simulink model "pacemaker_simulation"  (R2023b)
settings: Solver=FixedStepAuto  StartTime=0.0  StopTime=inf  FixedStep=1e-3  RelTol=1e-3  EnableMultiTasking=on
undefined symbols (not defined in the file): D0, D1, D10, D11, D12, D13, D2, D3, D4, D5, D6, D7, D8, D9, PTA0, PTA1, PTA2, PTB23, PTB9, PTC16, PTC17, PTC2, PTC3, PTC4, PTD0, PTD1, PTD2, PTD3
libraries: frdmk64flib x14
settings Model: ExtModeTrigDuration=5  Creator=stivb  LastModifiedBy=stivb
settings OptimizationCC: EnhancedBackFolding=on  PassReuseOutputArgsAs=Individual arguments  ZeroExternalMemoryAtStartup=off  ZeroInternalMemoryAtStartup=off  MaxStackSize=64  OptimizeBlockOrder=speed  DifferentSizesBufferReuse=on  OptimizationCustomize=off  EfficientTunableParamExpr=on
settings DebuggingCC: ParameterTunabilityLossMsg=error
settings HardwareCC: ProdBitPerPointer=32  ProdBitPerSizeT=32  ProdBitPerPtrDiffT=32  ProdLargestAtomicInteger=Long  ProdLargestAtomicFloat=Double  ProdWordSize=32  ProdHWDeviceType=ARM Compatible->ARM Cortex
settings SFSimCC: MATLABDynamicMemAlloc=off
settings RTWCC: Description=Embedded Coder  SystemTargetFile=ert.tlc  HardwareBoard=NXP FRDM-K64F  TLCOptions="-aInlineSetEventsForThisBaseRateFcn=TLC_FALSE -aSuppressMultiTaskScheduler=TLC_FALSE  -aRateBasedStepFcn=0"  TemplateMakefile=ert_default_tmf  Toolchain=GNU Tools for ARM Embedded Processors
settings CodeAppCC: ForceParamTrailComments=on  IgnoreCustomStorageClasses=off  OperatorAnnotations=on  SimulinkDataObjDesc=on  SFDataObjDesc=on  InsertBlockDesc=on
settings ERTTargetCC: ExtModeTransport=4  ExtModeMexFile=sendToCommService

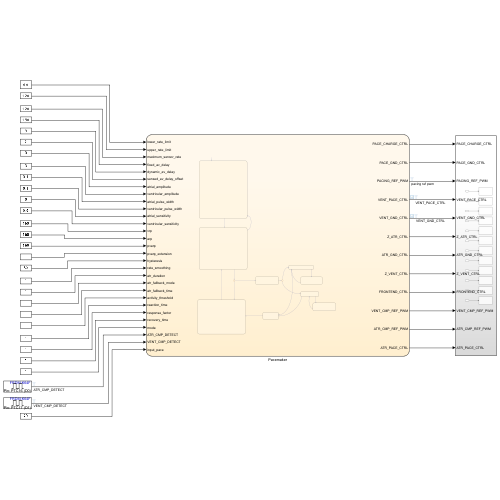
[thumbnail: Simulink's stored preview of the top-level diagram]
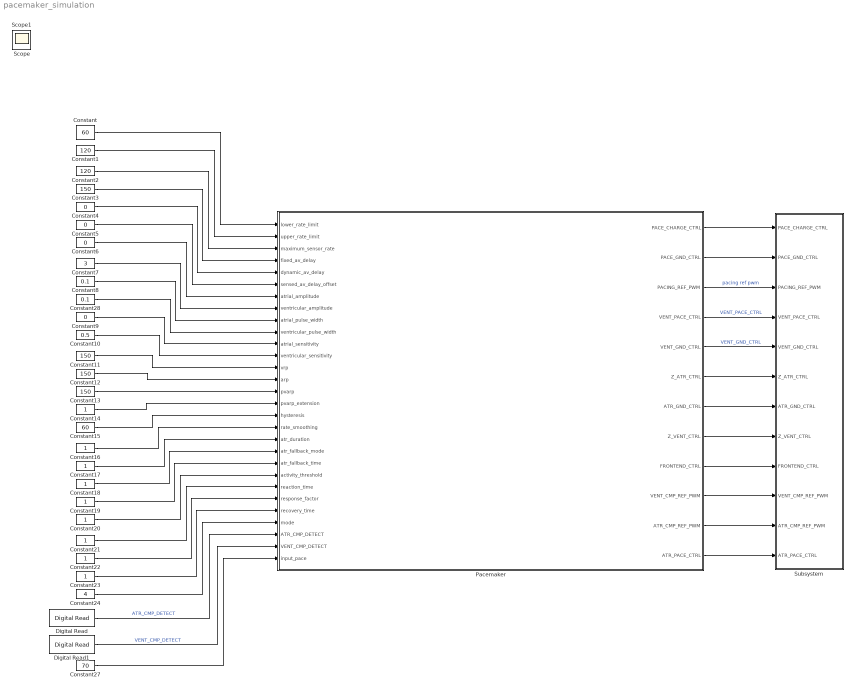
== system pacemaker_simulation ==
  Constant : Constant  Value=60
  Constant1 : Constant  Value=120
  Constant10 : Constant  Value=0.5
  Constant{3,11..13} (4 alike) : Constant  Value=150
  Constant{14,16..23} (9 alike) : Constant
  Constant15 : Constant  Value=60
  Constant2 : Constant  Value=120
  Constant24 : Constant  Value=4
  Constant27 : Constant  Value=70
  Constant28 : Constant  Value=0.1
  Constant{4..6,9} (4 alike) : Constant  Value=0
  Constant7 : Constant  Value=3
  Constant8 : Constant  Value=0.1
  Digital Read : frdmk64flib/Digital Read  Whichpin=PTC16 (D0)  SampleTime=-1
  Digital Read1 : frdmk64flib/Digital Read  Whichpin=PTC17 (D1)  SampleTime=-1
  Pacemaker : Stateflow chart  TreatAsAtomicUnit=on
      settings: PortSchema="{\"entries\":[{\"content\":{\"sides\":[{\"content\":{\"connectorIds\":[\"In1\",\"In2\",\"In3\",\"In4\",\"In5\",\"In6\",\"In7\",\"In8\",\"In9\",\"In10\",\"In11\",\"In12\",\"In13\",\"In14\",\"In15\",\"In16\",\"In17\",\"In18\",\"In19\",\"In20\",\"In21\",\"In22\",\"In23\",\"In24\",\"In25\",\"In29\",\"In26\",\"In27\",\"In28\"]},\"type\":\"ConnectorPlacement.EquallySpacedRectSide\",\"uuid\":\"0d0b6505-f176-4343-a9b1-ea9b59cb1490\"},{\"content\":{\"connectorIds\":[\"Out3\",\"Out4\",\"Out5\",\"Out6\",\"Out7\",\"Out8\",\"Out2\",\"Out9\",\"Out10\",\"Out11\",\"Out12\",\"Out1\"],\"side\":\"RIGHT\"},\"type\":\"ConnectorPlacement.EquallySpacedRectSide\",\"uuid\":\"eab01ff7-bf59-4a22-8f26-311ca37acfb7\"},{\"content\":{\"side\":\"TOP\"},\"type\":\"ConnectorPlacement.EquallySpacedRectSide\",\"uuid\":\"e74717db-4bd0-436d-8de4-c78dd455d9ac\"}]},\"type\":\"ConnectorPlacement.EquallySpacedConnector\",\"uuid\":\"6be528cb-4290-4782-81af-91f8ed75056e\"}],\"packageUris\":[\"http://schema.mathworks.com/mf0/Connector/R2020b\"],\"version\":\"1.0\"}"
  Subsystem : Subsystem
  Scope : Scope
  Scope1 : Scope
  wires:
  Constant/1 -> Pacemaker/1(lower_rate_limit)
  Constant10/1 -> Pacemaker/12(ventricular_sensitivity)
  Constant7/1 -> Pacemaker/8(ventricular_amplitude)
  Constant8/1 -> Pacemaker/9(atrial_pulse_width)
  Constant1/1 -> Pacemaker/2(upper_rate_limit)
  Constant6/1 -> Pacemaker/7(atrial_amplitude)
  Constant11/1 -> Pacemaker/13(vrp)
  Constant5/1 -> Pacemaker/6(sensed_av_delay_offset)
  Constant4/1 -> Pacemaker/5(dynamic_av_delay)
  Constant3/1 -> Pacemaker/4(fixed_av_delay)
  Constant2/1 -> Pacemaker/3(maximum_sensor_rate)
  Constant28/1 -> Pacemaker/10(ventricular_pulse_width)
  Pacemaker/7(VENT_GND_CTRL) -> Subsystem/5(VENT_GND_CTRL)  "VENT_GND_CTRL"
  Constant21/1 -> Pacemaker/23(reaction_time)
  Constant18/1 -> Pacemaker/20(atr_fallback_mode)
  Constant9/1 -> Pacemaker/11(atrial_sensitivity)
  Pacemaker/3(PACE_CHARGE_CTRL) -> Subsystem/1(PACE_CHARGE_CTRL)
  Constant15/1 -> Pacemaker/17(hysteresis)
  Constant12/1 -> Pacemaker/14(arp)
  Constant19/1 -> Pacemaker/21(atr_fallback_time)
  Constant16/1 -> Pacemaker/18(rate_smoothing)
  Constant13/1 -> Pacemaker/15(pvarp)
  Pacemaker/11(VENT_CMP_REF_PWM) -> Subsystem/10(VENT_CMP_REF_PWM)
  Constant20/1 -> Pacemaker/22(activity_threshold)
  Constant17/1 -> Pacemaker/19(atr_duration)
  Constant14/1 -> Pacemaker/16(pvarp_extension)
  Constant22/1 -> Pacemaker/24(response_factor)
  Constant23/1 -> Pacemaker/25(recovery_time)
  Constant24/1 -> Pacemaker/29(mode)
  Pacemaker/2(ATR_GND_CTRL) -> Subsystem/7(ATR_GND_CTRL)
  Digital Read/1 -> Pacemaker/26(ATR_CMP_DETECT)  "ATR_CMP_DETECT"
  Digital Read1/1 -> Pacemaker/27(VENT_CMP_DETECT)  "VENT_CMP_DETECT"
  Constant27/1 -> Pacemaker/28(input_pace)
  Pacemaker/4(PACE_GND_CTRL) -> Subsystem/2(PACE_GND_CTRL)
  Pacemaker/5(PACING_REF_PWM) -> Subsystem/3(PACING_REF_PWM)  "pacing ref pwm"
  Pacemaker/6(VENT_PACE_CTRL) -> Subsystem/4(VENT_PACE_CTRL)  "VENT_PACE_CTRL"
  Pacemaker/8(Z_ATR_CTRL) -> Subsystem/6(Z_ATR_CTRL)
  Pacemaker/9(Z_VENT_CTRL) -> Subsystem/8(Z_VENT_CTRL)
  Pacemaker/10(FRONTEND_CTRL) -> Subsystem/9(FRONTEND_CTRL)
  Pacemaker/12(ATR_CMP_REF_PWM) -> Subsystem/11(ATR_CMP_REF_PWM)
  Pacemaker/1(ATR_PACE_CTRL) -> Subsystem/12(ATR_PACE_CTRL)

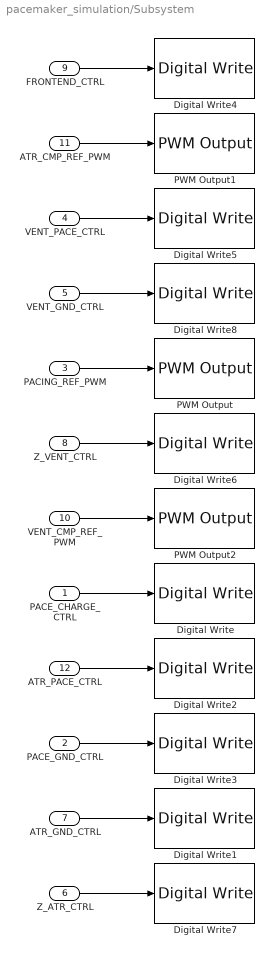
== system pacemaker_simulation/Subsystem ==
  PACE_CHARGE_CTRL : Inport
  PACE_GND_CTRL : Inport  Port=2
  PACING_REF_PWM : Inport  Port=3
  VENT_PACE_CTRL : Inport  Port=4
  VENT_GND_CTRL : Inport  Port=5
  Z_ATR_CTRL : Inport  Port=6
  ATR_GND_CTRL : Inport  Port=7
  Z_VENT_CTRL : Inport  Port=8
  FRONTEND_CTRL : Inport  Port=9
  VENT_CMP_REF_PWM : Inport  Port=10
  ATR_CMP_REF_PWM : Inport  Port=11
  ATR_PACE_CTRL : Inport  Port=12
  Digital Write : frdmk64flib/Digital Write  Whichpin=PTB9 (D2)
  Digital Write1 : frdmk64flib/Digital Write  Whichpin=PTD2 (D11)
  Digital Write2 : frdmk64flib/Digital Write  Whichpin=PTA0 (D8)
  Digital Write3 : frdmk64flib/Digital Write  Whichpin=PTD0 (D10)
  Digital Write4 : frdmk64flib/Digital Write  Whichpin=PTD1 (D13)
  Digital Write5 : frdmk64flib/Digital Write  Whichpin=PTC4 (D9)
  Digital Write6 : frdmk64flib/Digital Write  Whichpin=PTC3 (D7)
  Digital Write7 : frdmk64flib/Digital Write  Whichpin=PTB23 (D4)
  Digital Write8 : frdmk64flib/Digital Write  Whichpin=PTD3 (D12)
  PWM Output : frdmk64flib/PWM Output  Whichpin=PTA2 (D5)  InitialFrequency=2000  InitialDutyCycle=0
  PWM Output1 : frdmk64flib/PWM Output  Whichpin=PTC2 (D6)  InitialFrequency=2000  InitialDutyCycle=0
  PWM Output2 : frdmk64flib/PWM Output  Whichpin=PTA1 (D3)  InitialFrequency=2000  InitialDutyCycle=0
  wires:
  VENT_PACE_CTRL/1 -> Digital Write5/1
  Z_VENT_CTRL/1 -> Digital Write6/1
  PACE_CHARGE_CTRL/1 -> Digital Write/1
  Z_ATR_CTRL/1 -> Digital Write7/1
  PACING_REF_PWM/1 -> PWM Output/1
  ATR_GND_CTRL/1 -> Digital Write1/1
  ATR_CMP_REF_PWM/1 -> PWM Output1/1
  VENT_GND_CTRL/1 -> Digital Write8/1
  PACE_GND_CTRL/1 -> Digital Write3/1
  FRONTEND_CTRL/1 -> Digital Write4/1
  VENT_CMP_REF_PWM/1 -> PWM Output2/1
  ATR_PACE_CTRL/1 -> Digital Write2/1

== stateflow chart pacemaker_simulation/Pacemaker ==
  state Initalize
    if atrial_amplitude >0
    atrial_pacing =1;
    ventricle_pacing =0;
    pwm_threshold = atrial_amplitude/5;
    atrial_sensing = 1;
    ventricular_sensing = 0;
    pulse_width = atrial_pulse_width;
    ATR_CMP_REF_PWM = atrial_sensitivity/5; %mV
    else
    ventricle_pacing =1;
    atrial_pacing = 0;
    pwm_threshold = ventricular_amplitude/5;
    atrial_sensing = 0;
    ventricular_sensing = 1;
    pulse_width = ventricular_pulse_width;
    VENT_CMP_REF_PWM = ventricular_sensitivity/5;
    end
    if input_pace >= lower_rate_limit && input_pace <= upper_rate_limit
    automatic_interval = double((1/input_pace)*60*1000); %msec
    elseif (input_pace < lower_rate_limit)
    automatic_interval = double((1/lower_rate_limit)*60*1000); %msec
    else
    automatic_interval = double((1/upper_rate_limit)*60*1000); %msec
    end
    if hysteresis
    escape_interval = double((1/hysteresis)*60*1000);
    else
    escape_interval = automatic_interval; %sanity check
    end
    if(atrial_sensitivity>0 || ventricular_sensitivity > 0)
    is_sensing = 1;
    else
    is_sensing = 0;
    end
    previous_mode = mode;
  state Charge_Discharge_C22
    entry:
    %Charge
    ATR_PACE_CTRL = 0;
    VENT_PACE_CTRL = 0;
    PACE_CHARGE_CTRL = 1;
    PACING_REF_PWM = pwm_threshold; %percentage
    %Discharge
    PACE_GND_CTRL = 1;
    VENT_PACE_CTRL = 0;
    Z_ATR_CTRL = 0;
    Z_VENT_CTRL = 0;
    ATR_PACE_CTRL = 0;
    ATR_GND_CTRL = atrial_pacing;
    VENT_GND_CTRL= ventricle_pacing;
  state AtrialSensing
  note: Enter sensing state
  state EnterSensing
    entry:
    FRONTEND_CTRL = true;
    sensing_interval = automatic_interval;
  state AtrialEventDetected
    entry:
    sensing_interval = escape_interval;
  note: Set sensing interval to the escape interval since we are
      | using hysteresis pacing
  note: If not in sensing, continue pacing at automatic interval
  state VentricularSensing
  state ChargeC21
    %Creates the leading edge and sends pulse for X amount of time
    entry:
    PACE_CHARGE_CTRL = 0;
    PACE_GND_CTRL = 1;
    ATR_PACE_CTRL = atrial_pacing;
    ATR_GND_CTRL = 0;
    Z_ATR_CTRL = 0;
    Z_VENT_CTRL = 0;
    VENT_GND_CTRL = 0;
    VENT_PACE_CTRL = ventricle_pacing;
    %Recharge pulse is the current in the opposite direction due to C21
  state VentricularEventDetected
    entry:
    sensing_interval = escape_interval;
  state ExitSensing
    entry:
    FRONTEND_CTRL = false;
  (default) -> Initalize
  Charge_Discharge_C22 -> Initalize [order 2] : [hasChangedFrom(mode, previous_mode)]
  Initalize -> Charge_Discharge_C22
  (junction 100) -> AtrialSensing [order 1] : [atrial_sensing == 1 && after(arp, msec)]
  AtrialSensing -> ExitSensing [order 2] : [after(sensing_interval, msec)]
  AtrialEventDetected -> AtrialSensing : [after(arp, msec)]
  AtrialSensing -> AtrialEventDetected [order 1] : [hasChangedTo(ATR_CMP_DETECT, 1)]
  ChargeC21 -> Charge_Discharge_C22 : after(pulse_width, msec)
  Charge_Discharge_C22 -> (junction 106) [order 1]
  (junction 106) -> EnterSensing [order 2] : [is_sensing == 1]
  EnterSensing -> (junction 100)
  (junction 100) -> VentricularSensing [order 2] : [ventricular_sensing == 1 && after(vrp, msec)]
  (junction 106) -> ChargeC21 [order 1] : [is_sensing == 0 && after(automatic_interval, msec)]
  VentricularSensing -> ExitSensing [order 2] : [after(sensing_interval, msec)]
  VentricularEventDetected -> VentricularSensing : [after(vrp, msec)]
  VentricularSensing -> VentricularEventDetected [order 1] : [hasChangedTo(VENT_CMP_DETECT, 1)]
  ExitSensing -> ChargeC21
  data: ATR_PACE_CTRL output; ATR_GND_CTRL output; PACE_CHARGE_CTRL output; PACE_GND_CTRL output; PACING_REF_PWM output; VENT_PACE_CTRL output; VENT_GND_CTRL output; Z_ATR_CTRL output; Z_VENT_CTRL output; lower_rate_limit input; upper_rate_limit input; maximum_sensor_rate input; fixed_av_delay input; dynamic_av_delay input; sensed_av_delay_offset input; atrial_amplitude input; ventricular_amplitude input; atrial_pulse_width input; ventricular_pulse_width input; atrial_sensitivity input; ventricular_sensitivity input; vrp input; arp input; pvarp input; pvarp_extension input; hysteresis input; rate_smoothing input; atr_duration input; atr_fallback_mode input; atr_fallback_time input; activity_threshold input; reaction_time input; response_factor input; recovery_time input; FRONTEND_CTRL output boolean; ATR_CMP_DETECT input boolean; VENT_CMP_DETECT input boolean; sensing_interval local; atrial_pacing local; pulse_width local; pwm_threshold local; ventricle_pacing local; ventricular_sensing local; atrial_sensing local; VENT_CMP_REF_PWM output; ATR_CMP_REF_PWM output; automatic_interval local; escape_interval local; input_pace input; is_sensing local; mode input; previous_mode local
